simulink model "P6_S57_Totzeit"  (R2015a)
settings: Solver=ode45  StartTime=0.0  StopTime=500  RelTol=1e-3
settings Model: Creator=James  LastModifiedBy=James

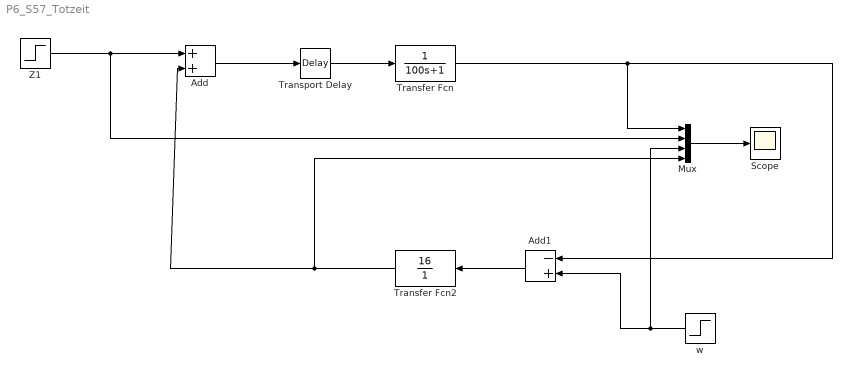
== system P6_S57_Totzeit ==
  Add : Sum
  Add1 : Sum  Inputs=-+
  Mux : Mux
  Scope : Scope
  Transfer Fcn : TransferFcn  Denominator=[100 1]
  Transfer Fcn2 : TransferFcn  Numerator=[16]  Denominator=[0 1]
  Transport Delay : TransportDelay  DelayTime=10
  "Z1 " : Step  Time=10  After=2
  "w " : Step  Time=300  After=2
  wires:
  "Z1 "/1 -> Mux/2, Add/1
  Transport Delay/1 -> Transfer Fcn/1
  Add/1 -> Transport Delay/1
  Transfer Fcn/1 -> Mux/1, Add1/1
  Mux/1 -> Scope/1
  Add1/1 -> Transfer Fcn2/1
  "w "/1 -> Mux/3, Add1/2
  Transfer Fcn2/1 -> Mux/4, Add/2
